simulink model "un_DTDSM_1b_2or_512osr"  (R2019b)
settings: Solver=VariableStepAuto  StartTime=0.0  StopTime=ts*(Mpoints+10)  RelTol=1e-3
InitFcn:
  | %fs=1024*2e4;
  | %osr=512;
  | ts=1/fs;
  | 
  | Ncycle=37;
  | Mpoints=2^16;
  | fin=fs*Ncycle/Mpoints;
  | 
  | 
  | ref=2;
values from neighbouring files (symbols this model uses):
  fs = osr*2*2e4    (= 40960000)    [CTSDM.m]
  osr = 1024    [CTSDM.m]    (also in ENOB.m = logspace(log10(64), log10(2^15), 1000); SNR.m = logspace(log10(64), log10(2^15), 1000))
undefined symbols (not defined in the file or in its folder): a1, argo, b1, c1
libraries: SDtoolbox x2
settings Model: Creator=lenovo  LastModifiedBy=lenovo

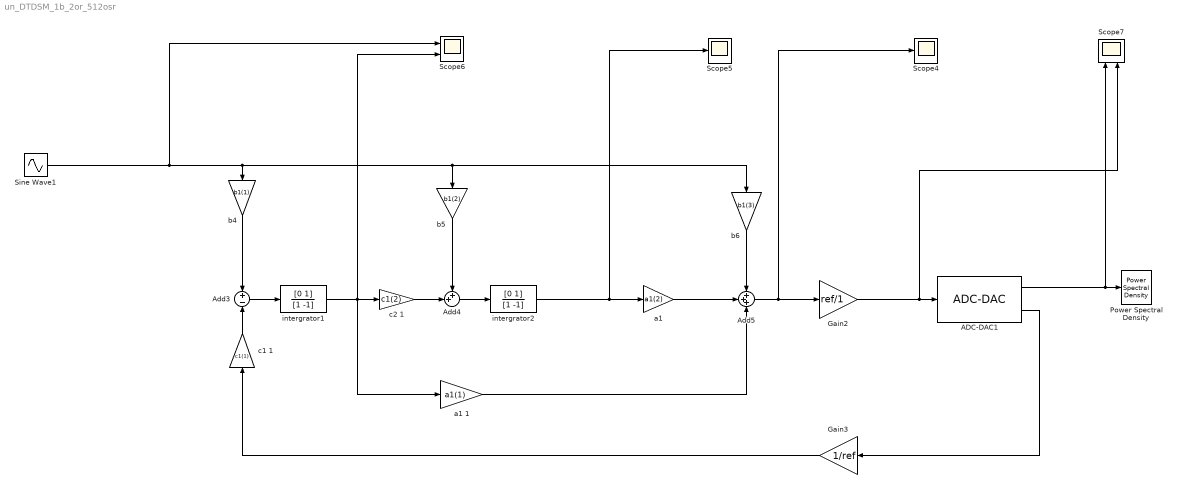
== system un_DTDSM_1b_2or_512osr ==
  ADC-DAC1 : SDtoolbox/ADC-DAC  k=1  MM=off  match=0  CST=0  VVG=off  argo=argo(:,3)  LF=on  NF=retA.log
      settings: SourceProductName=SDtoolbox
  Add3 : Sum  Inputs=+|-
  Add4 : Sum  Inputs=++|
  Add5 : Sum  Inputs=+++
  Gain2 : Gain  Gain=ref/1
  Gain3 : Gain  Gain=1/ref
  Power Spectral Density : SDtoolbox/Power Spectral Density  SN=2  Fs=fs  fBL=1  fBH=fs/(2*osr)  Fin=fin  N=Mpoints  Ntransient=10  VW=on  savename=1  Scale_type=logarithmic
      settings: SourceProductName=SDtoolbox
  Scope4 : Scope
  Scope5 : Scope
  Scope6 : Scope  NumInputPorts=2
  Scope7 : Scope  NumInputPorts=2
  Sine Wave1 : Sin  Amplitude=0.435  Frequency=fin*2*pi  SampleTime=ts
  a1 : Gain  Gain=a1(2)
  a1 1 : Gain  Gain=a1(1)
  b4 : Gain  Gain=b1(1)
  b5 : Gain  Gain=b1(2)
  b6 : Gain  Gain=b1(3)
  c1 1 : Gain  Gain=c1(1)
  c2 1 : Gain  Gain=c1(2)
  intergrator1 : DiscreteFilter  Numerator=[0 1]  Denominator=[1 -1]
  intergrator2 : DiscreteFilter  Numerator=[0 1]  Denominator=[1 -1]
  wires:
  c2 1/1 -> Add4/2
  Gain2/1 -> ADC-DAC1/1, Scope7/2
  ADC-DAC1/1 -> Power Spectral Density/1, Scope7/1
  Add5/1 -> Scope4/1, Gain2/1
  ADC-DAC1/2 -> Gain3/1
  b4/1 -> Add3/1
  b6/1 -> Add5/1
  a1/1 -> Add5/2
  c1 1/1 -> Add3/2
  intergrator1/1 -> Scope6/2, a1 1/1, c2 1/1
  b5/1 -> Add4/1
  Gain3/1 -> c1 1/1
  a1 1/1 -> Add5/3
  intergrator2/1 -> Scope5/1, a1/1
  Add3/1 -> intergrator1/1
  Add4/1 -> intergrator2/1
  Sine Wave1/1 -> Scope6/1, b6/1, b5/1, b4/1
